simulink model "Battery_Thevenin_Model_RC"  (R2025b)
settings: Solver=ode1  StartTime=0.0  StopTime=Ttotal  FixedStep=Tsample  MaxStep=1e-3  RelTol=1e-3
values from neighbouring files (symbols this model uses):
  C_nom = 90    [Battery_Parameters_RC.m]
  C_total = C_nom*3600    (= 324000)    [Battery_Parameters_RC.m]
settings Model: Creator=mwxiao  LastModifiedBy=carter
settings SolverCC: AlgebraicLoopSolver=TrustRegion
settings DataIOCC: LimitDataPoints=on  SaveFormat=Array  SignalLoggingSaveFormat=ModelDataLogs  ReturnWorkspaceOutputs=off  SignalLoggingName=sigsOut
settings OptimizationCC: ExpressionDepthLimit=2147483647.0  LifeSpan=inf
settings DebuggingCC: SaveWithParameterizedLinksMsg=none  UnderspecifiedInitializationDetection=Classic  MergeDetectMultiDrivingBlocksExec=none  SignalResolutionControl=TryResolveAllWithWarning  MultiTaskDSMMsg=warning  MultiTaskCondExecSysMsg=none  FcnCallInpInsideContextMsg=warning  UnconnectedInputMsg=warning  UnconnectedOutputMsg=warning  UnconnectedLineMsg=warning  StateNameClashWarn=warning  SFUnexpectedBacktrackingDiag=warning  SFNoUnconditionalDefaultTransitionDiag=warning  SFExecutionAtInitializationDiag=none  ArithmeticOperatorsInVariantConditions=warning
settings HardwareCC: ProdBitPerPointer=32.0  ProdBitPerSizeT=32.0  ProdBitPerPtrDiffT=32.0  ProdLargestAtomicFloat=None  ProdIntDivRoundTo=Undefined  ProdEndianess=Unspecified  ProdWordSize=32.0  ProdHWDeviceType=32-bit Generic  TargetUnknown=on
settings ModelReferenceCC: EnableRefExpFcnMdlSchedulingChecks=on  PropagateSignalLabelsOutOfModel=off
settings SFSimCC: SimUseLocalCustomCode=off  CustomCodeUndefinedFunction=UseInterfaceOnly
settings RTWCC: RTWUseLocalCustomCode=off  GPUComputeCapability=3.5  DLArmComputeVersion=19.05
settings CodeAppCC: StateflowObjectComments=on
settings GRTTargetCC: TargetLangStandard=C89/C90 (ANSI)  CombineOutputUpdateFcns=off  GRTInterface=on
settings ConfigComp: CovMetricSettings=dw  CovSaveCumulativeToWorkspaceVar=on  CovSaveSingleToWorkspaceVar=on  CovExternalEMLEnable=off

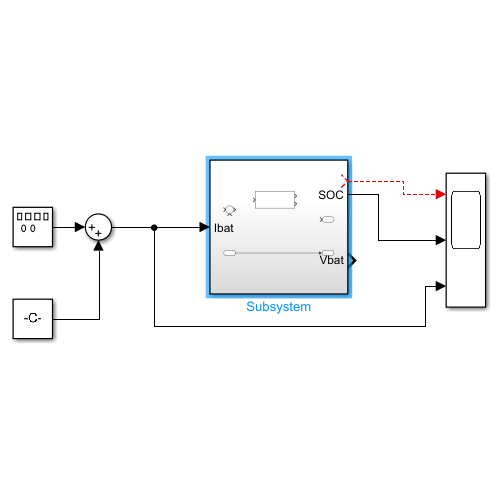
[thumbnail: Simulink's stored preview of the top-level diagram]
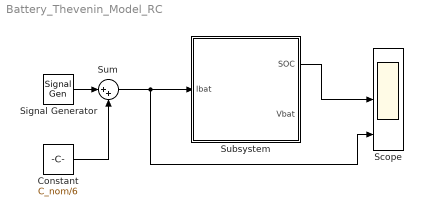
== system Battery_Thevenin_Model_RC ==
  Constant : Constant  Value=C_nom/6
  Scope : Scope  NumInputPorts=3
  Signal Generator : SignalGenerator  Units=rad/sec
  Subsystem : Subsystem
  Sum : Sum  Inputs=|++
  wires:
  Signal Generator/1 -> Sum/1
  Sum/1 -> Scope/3, Subsystem/1(Ibat)
  Constant/1 -> Sum/2
  ? -> Scope/1
  Subsystem/1(SOC) -> Scope/2

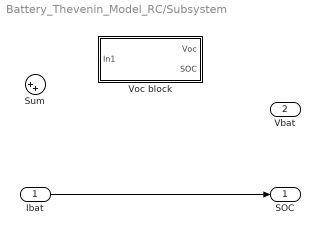
== system Battery_Thevenin_Model_RC/Subsystem ==
  Ibat : Inport
  Sum : Sum  Inputs=|++
  Voc block : Subsystem
  SOC : Outport
  Vbat : Outport  Port=2
  wires:
  Ibat/1 -> SOC/1

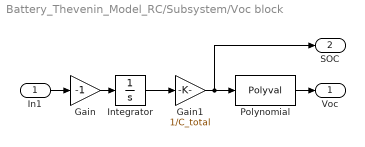
== system Battery_Thevenin_Model_RC/Subsystem/Voc block ==
  In1 : Inport
  Gain : Gain  Gain=-1
  Gain1 : Gain  Gain=1/C_total
  Integrator : Integrator  LimitOutput=on  LowerSaturationLimit=0
  Polynomial : Polyval  Coefs=[ +2.081618890e-019, -1.441693666e-014, +4.719686976e-010, -8.536869453e-006, +1.621573104e-001, -8.087801117e+001 ]
  Voc : Outport
  SOC : Outport  Port=2
  wires:
  In1/1 -> Gain/1
  Gain/1 -> Integrator/1
  Polynomial/1 -> Voc/1
  Integrator/1 -> Gain1/1
  Gain1/1 -> SOC/1, Polynomial/1
